simulink model "analog_bp_3"  (Simulink 7.7)
settings: Solver=ode45  StartTime=0.0  StopTime=100e-3  MaxStep=1e-6  RelTol=1e-3
values from neighbouring files (symbols this model uses):
  a = zeros(5, nord+1)    [analog_tp1.m]    (also in analog_tp2.m)
  b = fir1(nr-1,0.5)    [adapt_filter1.m]    (also in adapt_filter2.m; analog_tp1.m = zeros(5, nord+1); analog_tp2.m = zeros(5, nord+1))
  f1s = 30100    [analog_bp3.m]
  f2s = 30400    [analog_bp3.m]
  frausch = 250    [analog_bp3.m]    (also in analog_tp2.m = 500)
  k1 = 0    [analog_bp3.m]
  k2 = 1    [analog_bp3.m]
  k3 = 1    [analog_bp3.m]
  k4 = 0    [analog_bp3.m]
libraries: dsparch4 x1
settings Model: Creator=svenhoffmann  LastModifiedBy=josef  ExtModeAutoUpdateStatusClock=off
settings DataIOCC: LimitDataPoints=off  SignalLoggingName=sigsOut
settings DebuggingCC: SaveWithParameterizedLinksMsg=none  SignalResolutionControl=TryResolveAllWithWarning  SolverPrmCheckMsg=none  MultiTaskDSMMsg=warning  MultiTaskCondExecSysMsg=none  StrictBusMsg=None
settings HardwareCC: TargetUnknown=on
settings RTWCC: IncludeERTFirstTime=on

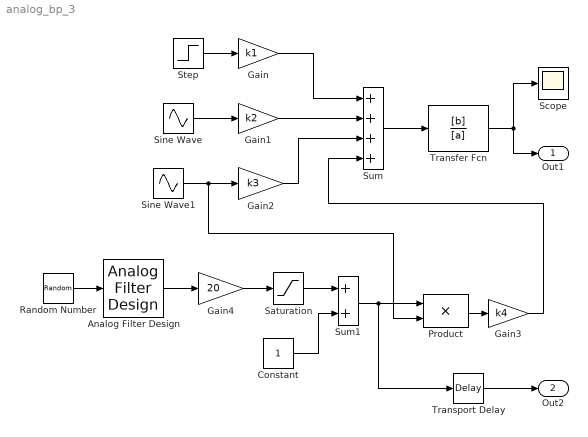
== system analog_bp_3 ==
  Analog Filter Design : dsparch4/Analog Filter Design  method=Chebyshev I  filttype=Lowpass  N=8  Wlo=2*pi*frausch  Whi=80  Rp=1  Rs=60
  Constant : Constant
  Gain : Gain  Gain=k1  SaturateOnIntegerOverflow=on  OutDataTypeStr=Inherit: Same as input  ParamDataTypeStr=Inherit: Same as input
  Gain1 : Gain  Gain=k2  SaturateOnIntegerOverflow=on  OutDataTypeStr=Inherit: Same as input  ParamDataTypeStr=Inherit: Same as input
  Gain2 : Gain  Gain=k3  SaturateOnIntegerOverflow=on  OutDataTypeStr=Inherit: Same as input  ParamDataTypeStr=Inherit: Same as input
  Gain3 : Gain  Gain=k4  SaturateOnIntegerOverflow=on  OutDataTypeStr=Inherit: Same as input  ParamDataTypeStr=Inherit: Same as input
  Gain4 : Gain  Gain=20  SaturateOnIntegerOverflow=on  OutDataTypeStr=Inherit: Same as input  ParamDataTypeStr=Inherit: Same as input
  Product : Product  SaturateOnIntegerOverflow=on  OutDataTypeStr=Inherit: Same as first input
  Random Number : RandomNumber  SampleTime=0
  Saturation : Saturate  UpperLimit=1  LowerLimit=-1
  Scope : Scope
  Sine Wave : Sin  Frequency=2*pi*f1s  SampleTime=0
  Sine Wave1 : Sin  Frequency=2*pi*f2s  SampleTime=0
  Step : Step  Time=0  SampleTime=0
  Sum : Sum  Inputs=++++  SaturateOnIntegerOverflow=on
  Sum1 : Sum  SaturateOnIntegerOverflow=on
  Transfer Fcn : TransferFcn  Numerator=[b]  Denominator=[a]
  Transport Delay : TransportDelay  DelayTime=1.5e-3  BufferSize=2048
  Out1 : Outport
  Out2 : Outport  Port=2
  wires:
  Random Number/1 -> Analog Filter Design/1
  Step/1 -> Gain/1
  Sine Wave/1 -> Gain1/1
  Sine Wave1/1 -> Gain2/1, Product/2
  Gain1/1 -> Sum/2
  Gain2/1 -> Sum/3
  Gain3/1 -> Sum/4
  Sum/1 -> Transfer Fcn/1
  Transfer Fcn/1 -> Scope/1, Out1/1
  Product/1 -> Gain3/1
  Analog Filter Design/1 -> Gain4/1
  Sum1/1 -> Product/1, Transport Delay/1
  Gain4/1 -> Saturation/1
  Saturation/1 -> Sum1/1
  Transport Delay/1 -> Out2/1
  Gain/1 -> Sum/1
  Constant/1 -> Sum1/2
